simulink model "Led_Stateflow_App"  (R2024a)
settings: Solver=VariableStepAuto  StartTime=0.0  StopTime=10.0  RelTol=1e-3
settings Model: Creator=DELL  LastModifiedBy=DELL

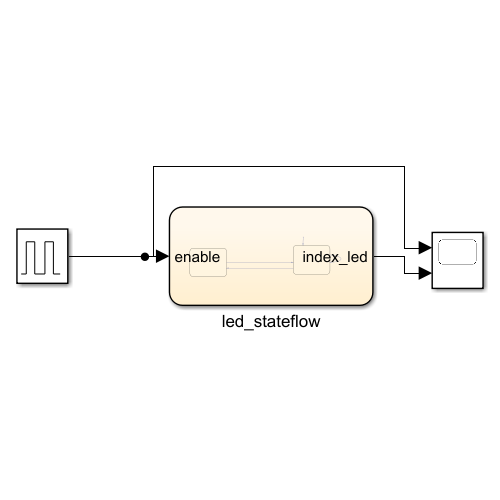
[thumbnail: Simulink's stored preview of the top-level diagram]
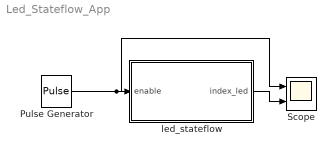
== system Led_Stateflow_App ==
  Pulse Generator : DiscretePulseGenerator  PulseType=Time based  PulseWidth=50
  Scope : Scope  NumInputPorts=2
  led_stateflow : Stateflow chart  TreatAsAtomicUnit=on
  wires:
  led_stateflow/1(index_led) -> Scope/2
  Pulse Generator/1 -> Scope/1, led_stateflow/1(enable)

== stateflow chart Led_Stateflow_App/led_stateflow ==
  state LedOff
    entry:
    index_led=0;
  state LedOn
    entry:
    index_led=1;
  (default) -> LedOff
  LedOff -> LedOff [order 2] : [enable==0]
  LedOn -> LedOff : after(1,tick)
  LedOff -> LedOn [order 1] : after(1,tick)[enable==1]
  data: index_led output; enable input
